simulink model "P1_sim"  (R2020b)
settings: Solver=FixedStepAuto  StartTime=0.0  StopTime=25  FixedStep=0.001  RelTol=1e-3
model workspace (MAT data in the model file):
  eslasticidade = 0
  teste = 0
libraries: simulink x1
settings Model: Creator=Tiago  LastModifiedBy=Tiago
settings SolverCC: ZeroCrossAlgorithm=Adaptive
settings DataIOCC: SaveState=on
settings DebuggingCC: IgnoredZcDiagnostic=none

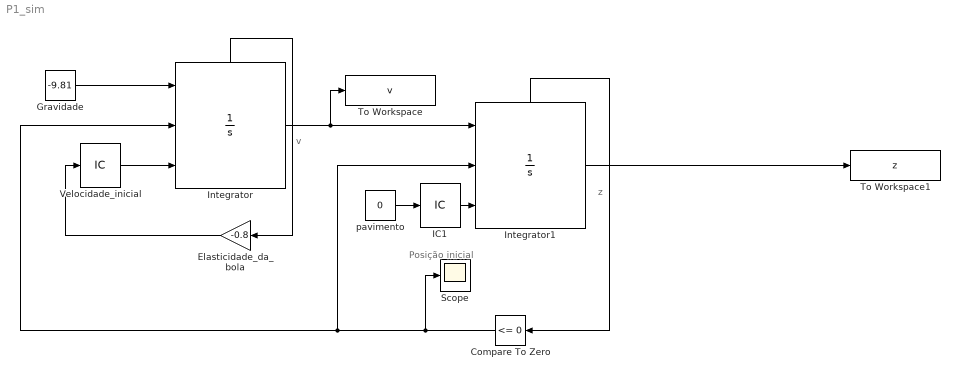
== system P1_sim ==
  note: Posição inicial
  note: z
  note: v
  Compare To Zero : simulink/Logic and Bit Operations/Compare To Zero  relop=<=  OutDataTypeStr=boolean
  Elasticidade_da_bola : Gain  Tag=teste  Gain=-0.8
  Gravidade : Constant  Value=-9.81
  IC1 : InitialCondition  Value=10
  Integrator : Integrator  ExternalReset=rising  InitialConditionSource=external  ShowStatePort=on
  Integrator1 : Integrator  ExternalReset=rising  InitialConditionSource=external  ShowStatePort=on
  Scope : Scope
  To Workspace : ToWorkspace  VariableName=v  SaveFormat=Timeseries  SampleTime=-1
  To Workspace1 : ToWorkspace  VariableName=z  SaveFormat=Timeseries  SampleTime=-1
  Velocidade_inicial : InitialCondition  Value=5
  pavimento : Constant  Value=0
  wires:
  Gravidade/1 -> Integrator/1
  Velocidade_inicial/1 -> Integrator/3
  Integrator/State -> Elasticidade_da_bola/1
  Integrator/1 -> To Workspace/1, Integrator1/1
  IC1/1 -> Integrator1/3
  pavimento/1 -> IC1/1
  Integrator1/State -> Compare To Zero/1
  Compare To Zero/1 -> Integrator/2, Integrator1/2, Scope/1
  Integrator1/1 -> To Workspace1/1
  Elasticidade_da_bola/1 -> Velocidade_inicial/1
